simulink model "Task18"  (R2025a)
settings: Solver=VariableStepAuto  StartTime=0.0  StopTime=10.0  RelTol=1e-3
libraries: simulink x1
settings Model: Creator=LOQ  LastModifiedBy=LOQ

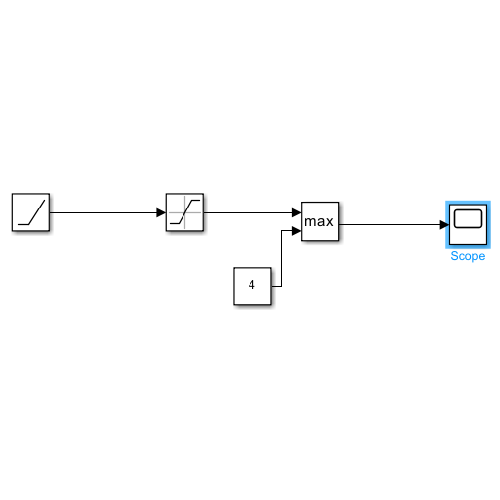
[thumbnail: Simulink's stored preview of the top-level diagram]
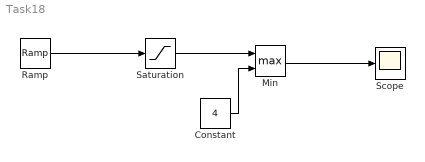
== system Task18 ==
  Constant : Constant  Value=4
  Min : MinMax  Function=max  Inputs=2
  Ramp : simulink/Sources/Ramp  slope=2  start=0  InitialOutput=0
  Saturation : Saturate  UpperLimit=10  LowerLimit=0
  Scope : Scope
      settings: ActiveDisplayYMinimum=3.25  ActiveDisplayYMaximum=10.75
  wires:
  Ramp/1 -> Saturation/1
  Constant/1 -> Min/2
  Saturation/1 -> Min/1
  Min/1 -> Scope/1
